simulink model "mymodel"  (R2023b)
settings: Solver=ode4  StartTime=0.0  StopTime=inf  FixedStep=0.01  RelTol=1e-3
values from neighbouring files (symbols this model uses):
  b = 10    [workspaceInit.mat]
  k = 400    [workspaceInit.mat]
  m = 3.6    [workspaceInit.mat]
undefined symbols (not defined in the file or in its folder): DiscIntNeverNeededParam
settings Model: Creator=cigla  LastModifiedBy=cigla
settings OptimizationCC: EnhancedBackFolding=on  PassReuseOutputArgsAs=Individual arguments  ZeroExternalMemoryAtStartup=off  ZeroInternalMemoryAtStartup=off  OptimizeBlockOrder=speed  DifferentSizesBufferReuse=on  OptimizationCustomize=off  EfficientTunableParamExpr=on
settings DebuggingCC: ParameterTunabilityLossMsg=error
settings SFSimCC: MATLABDynamicMemAlloc=off
settings RTWCC: Description=Embedded Coder  SystemTargetFile=ert.tlc  TemplateMakefile=ert_default_tmf  BuildConfiguration=Debug
settings CodeAppCC: ForceParamTrailComments=on  IgnoreCustomStorageClasses=off  OperatorAnnotations=on  SimulinkDataObjDesc=on  SFDataObjDesc=on  InsertBlockDesc=on
settings ERTTargetCC: TargetLangStandard=C99 (ISO)  GenerateSampleERTMain=on  ERTCustomFileTemplate=example_file_process.tlc

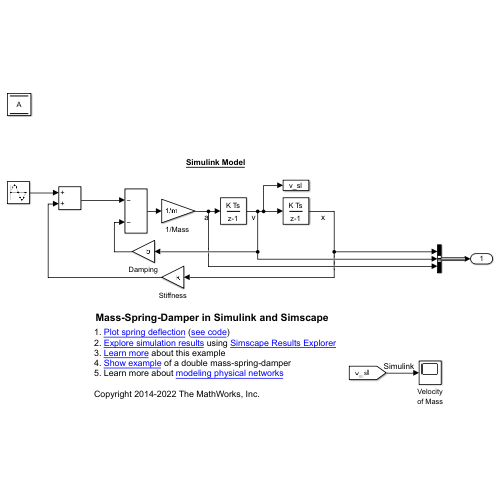
[thumbnail: Simulink's stored preview of the top-level diagram]
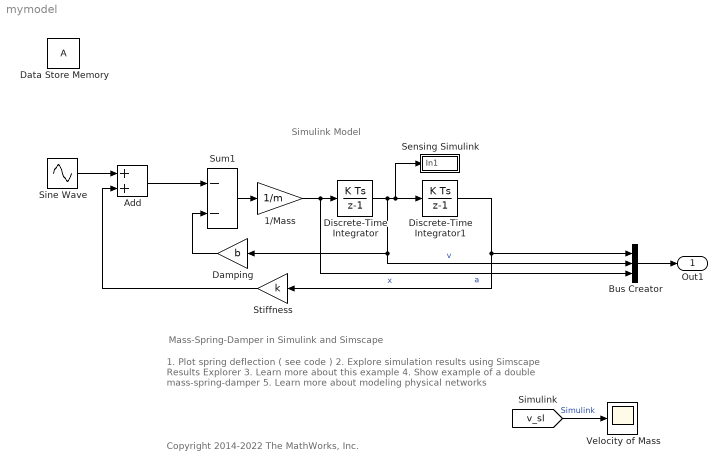
== system mymodel ==
  note: Simulink Model
  note: 1. Plot spring deflection ( see code )
      | 2. Explore simulation results using Simscape Results Explorer
      | 3. Learn more about this example
      | 4. Show example of a double mass-spring-damper
      | 5. Learn more about modeling physical networks
  note: Mass-Spring-Damper in Simulink and Simscape
  note: Copyright 2014-2022 The MathWorks, Inc.
  "1/Mass " : Gain  Gain=1/m  SaturateOnIntegerOverflow=on  OutDataTypeStr=Inherit: Same as input  ParamDataTypeStr=Inherit: Same as input
  Add : Sum
  Bus Creator : BusCreator  Inputs=3
  Damping : Gain  Gain=b  SaturateOnIntegerOverflow=on  OutDataTypeStr=Inherit: Same as input  ParamDataTypeStr=Inherit: Same as input
  Data Store Memory : DataStoreMemory  WriteAfterWriteMsg=warning  ShowAdditionalParam=off
  Discrete-Time Integrator : DiscreteIntegrator  SampleTime=-1  ICPrevOutput=DiscIntNeverNeededParam  ICPrevScaledInput=DiscIntNeverNeededParam
  Discrete-Time Integrator1 : DiscreteIntegrator  SampleTime=-1  ICPrevOutput=DiscIntNeverNeededParam  ICPrevScaledInput=DiscIntNeverNeededParam
  Sensing Simulink : Subsystem
      mask Display: disp('v_sl')
  Sine Wave : Sin  SineType=Sample based  Amplitude=10  Frequency=10  SampleTime=0.01
  Stiffness : Gain  Gain=k  SaturateOnIntegerOverflow=on  OutDataTypeStr=Inherit: Same as input  ParamDataTypeStr=Inherit: Same as input
  Sum1 : Sum  Inputs=--  InputSameDT=on  SaturateOnIntegerOverflow=on  OutDataTypeStr=Inherit: Same as first input
  Velocity of Mass : Scope
  Out1 : Outport
  wires:
  Discrete-Time Integrator1/1 -> Stiffness/1, Bus Creator/1  "x"
  [v_sl] -> Velocity of Mass/1  "Simulink"
  Discrete-Time Integrator/1 -> Sensing Simulink/1(In1), Discrete-Time Integrator1/1, Bus Creator/2, Damping/1  "v"
  "1/Mass "/1 -> Bus Creator/3, Discrete-Time Integrator/1  "a"
  Stiffness/1 -> Add/2
  Damping/1 -> Sum1/2
  Sum1/1 -> "1/Mass "/1
  Add/1 -> Sum1/1
  Sine Wave/1 -> Add/1
  Bus Creator/1 -> Out1/1

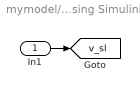
== system mymodel/Sensing Simulink ==
  In1 : Inport
  tag scope: v_sl=global
  wires:
  In1/1 -> [v_sl]
